simulink model "sim_implicit_IC_nonlinear"  (R2017b)
settings: Solver=VariableStepAuto  StartTime=0.0  StopTime=10.0  RelTol=1e-3
values from neighbouring files (symbols this model uses):
  g = 9.81    [init_sim.m]
  InvSet_phiA = InvSet_phi.A    [init_sim.m]
  InvSet_phib = InvSet_phi.b    [init_sim.m]
  InvSet_yA = InvSet_y.A    [init_sim.m]
  InvSet_yb = InvSet_y.b    [init_sim.m]
  InvSet_zA = InvSet_z.A    [init_sim.m]
  InvSet_zb = InvSet_z.b    [init_sim.m]
  LQRSet_phiA = LQRSet_phi.A    [init_sim.m]
  LQRSet_phib = LQRSet_phi.b    [init_sim.m]
  LQRSet_yA = LQRSet_y.A    [init_sim.m]
  LQRSet_yb = LQRSet_y.b    [init_sim.m]
  LQRSet_zA = LQRSet_z.A    [init_sim.m]
  LQRSet_zb = LQRSet_z.b    [init_sim.m]
  u_max = [f_max; tau_max]    [init_sim.m]
  u_min = [f_min; tau_min]    [init_sim.m]
  x0 = zeros(6,1)    [get_sim_data.m]    (also in get_sim_data_mpc_phi.m; get_sim_data_mpc_y.m; get_sim_data_mpc_z.m; init_sim.m = 0.9*[InvSet_y.V(i,1)'; InvSet_z.V(j,1)'; InvSet_phi.V(k,1)';)
  x_max = [y_max;z_max;angle_max;vy_max;vz_max;arate_max]    [init_sim.m]
  x_min = [y_min;z_min;angle_min;vy_min;vz_min;arate_min]    [init_sim.m]
undefined symbols (not defined in the file or in its folder): K_phi, K_y, K_z, uavPlanarNonlin
settings Model: Creator=zboucek  LastModifiedBy=zboucek

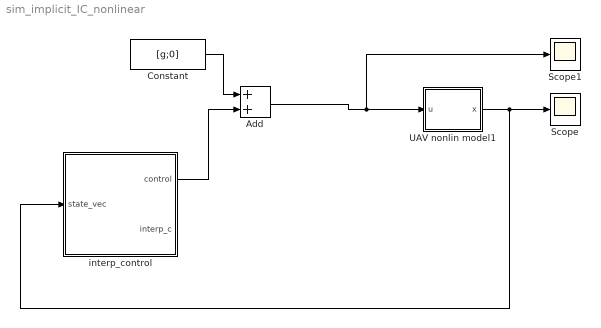
== system sim_implicit_IC_nonlinear ==
  Add : Sum
  Constant : Constant  Value=[g;0]  VectorParams1D=off
  Scope : Scope
  Scope1 : Scope
  UAV nonlin model1 : Subsystem
  interp_control : MATLAB Function  TreatAsAtomicUnit=on
  wires:
  UAV nonlin model1/1(x) -> interp_control/1(state_vec), Scope/1
  interp_control/1(control) -> Add/2
  Add/1 -> UAV nonlin model1/1(u), Scope1/1
  Constant/1 -> Add/1

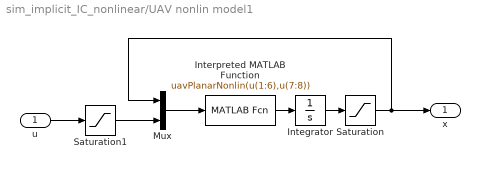
== system sim_implicit_IC_nonlinear/UAV nonlin model1 ==
  u : Inport
  Integrator : Integrator  InitialCondition=x0
  Interpreted MATLAB Function : MATLABFcn  MATLABFcn=uavPlanarNonlin(u(1:6),u(7:8))  OutputDimensions=6
  Mux : Mux  Inputs=2
  Saturation : Saturate  UpperLimit=x_max  LowerLimit=x_min
  Saturation1 : Saturate  UpperLimit=u_max  LowerLimit=u_min
  x : Outport
  wires:
  Mux/1 -> Interpreted MATLAB Function/1
  Interpreted MATLAB Function/1 -> Integrator/1
  Integrator/1 -> Saturation/1
  Saturation/1 -> x/1, Mux/1
  u/1 -> Saturation1/1
  Saturation1/1 -> Mux/2

== matlab function sim_implicit_IC_nonlinear/interp_control ==
  settings: updateMethod=DISCRETE  sampleTime=Ts
  data: state_vec input; control output; interp_c output; InvSet_yA parameter; InvSet_zA parameter; LQRSet_phiA parameter; LQRSet_yA parameter; LQRSet_zA parameter; InvSet_phiA parameter; K_y parameter; K_z parameter; K_phi parameter; InvSet_phib parameter; InvSet_yb parameter; InvSet_zb parameter; LQRSet_phib parameter; LQRSet_yb parameter; LQRSet_zb parameter
function [control,interp_c]= interpolation(state_vec, InvSet_yA, InvSet_zA, LQRSet_phiA, LQRSet_yA, LQRSet_zA, InvSet_phiA, K_y, K_z, K_phi, InvSet_phib, InvSet_yb, InvSet_zb, LQRSet_phib, LQRSet_yb, LQRSet_zb)

% optimization variables
c = sdpvar(1, 1);
rv = sdpvar(2,1);
J = c;


x = state_vec([1,4]);
C = [InvSet_yA*rv <= c*InvSet_yb; LQRSet_yA*(x'-rv) <= (1-c)*LQRSet_yb; 0 <= c <= 1];
% options = sdpsettings('solver','linprog','verbose',0,'cachesolvers',1);  % setup LP-solver  
% optimize(C, J, options);
optimize(C, J);
rvk = value(rv);
r0 = x' - rvk;
uvk=quad_vertex_y(rvk);
u_y = K_y*r0 + uvk(1:1,1);
cval_y = value(c);

x = state_vec([2,5]);
C = [InvSet_zA*rv <= c*InvSet_zb; LQRSet_zA*(x'-rv) <= (1-c)*LQRSet_zb; 0 <= c <= 1];
% options = sdpsettings('solver','linprog','verbose',0,'cachesolvers',1);  % setup LP-solver  
% optimize(C, J, options);
optimize(C, J);
rvk = value(rv);
r0 = x' - rvk;
uvk=quad_vertex_z(rvk);
u_z = K_z*r0 + uvk(1:1,1);
cval_z = value(c);

x = state_vec([3,6])-[u_y;0];
C = [InvSet_phiA*rv <= c*InvSet_phib; LQRSet_phiA*(x'-rv) <= (1-c)*LQRSet_phib; 0 <= c <= 1];
% options = sdpsettings('solver','linprog','verbose',0,'cachesolvers',1);  % setup LP-solver  
% optimize(C, J, options);
optimize(C, J);
rvk = value(rv);
r0 = x' - rvk;
uvk=quad_vertex_phi(rvk);
u_phi = K_phi*r0 + uvk(1:1,1);
cval_phi = value(c);

control = [u_z;u_phi];
interp_c = [cval_y;cval_z;cval_phi];
